simulink model "Astatic_StateSpace"  (R2021a)
settings: Solver=FixedStepAuto  StartTime=0.0  StopTime=STime  FixedStep=1e-3  RelTol=1e-3
undefined symbols (not defined in the file): C, J, Ka_, Kp, Mc, Ra, Ta, Tp, TPert
settings Model: Creator=akangmufti  LastModifiedBy=akangmufti

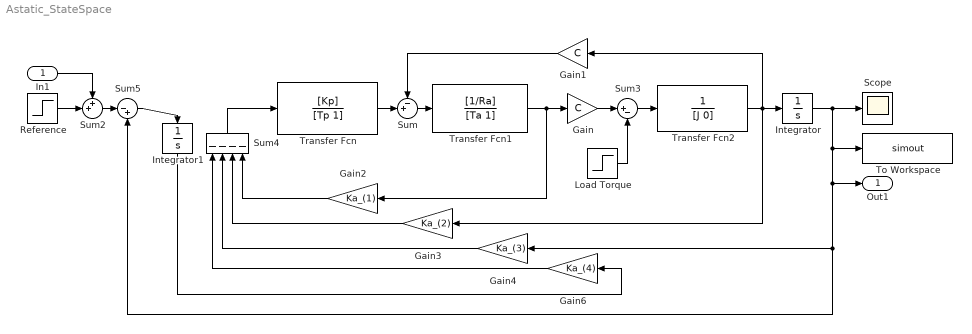
== system Astatic_StateSpace ==
  In1 : Inport
  Gain : Gain  Gain=C
  Gain1 : Gain  Gain=C
  Gain2 : Gain  Gain=Ka_(1)
  Gain3 : Gain  Gain=Ka_(2)
  Gain4 : Gain  Gain=Ka_(3)
  Gain6 : Gain  Gain=Ka_(4)
  Integrator : Integrator
  Integrator1 : Integrator
  Load Torque : Step  Time=TPert  After=Mc  SampleTime=0
  Reference : Step  Time=1e-3  SampleTime=0
  Scope : Scope
  Sum : Sum  Inputs=-+|
  Sum2 : Sum  Inputs=++|
  Sum3 : Sum  Inputs=|+-
  Sum4 : Sum  Inputs=----
  Sum5 : Sum  Inputs=|-+
  To Workspace : ToWorkspace  VariableName=simout  SampleTime=-1
  Transfer Fcn : TransferFcn  Numerator=[Kp]  Denominator=[Tp 1]
  Transfer Fcn1 : TransferFcn  Numerator=[1/Ra]  Denominator=[Ta 1]
  Transfer Fcn2 : TransferFcn  Denominator=[J 0]
  Out1 : Outport
  wires:
  Gain/1 -> Sum3/1
  Sum/1 -> Transfer Fcn1/1
  Transfer Fcn1/1 -> Gain2/1, Gain/1
  Transfer Fcn/1 -> Sum/2
  Gain1/1 -> Sum/1
  Sum3/1 -> Transfer Fcn2/1
  Transfer Fcn2/1 -> Gain3/1, Integrator/1, Gain1/1
  Load Torque/1 -> Sum3/2
  Gain3/1 -> Sum4/3
  Gain4/1 -> Sum4/2
  Gain2/1 -> Sum4/4
  Sum4/1 -> Transfer Fcn/1
  Integrator1/1 -> Gain6/1
  Sum5/1 -> Integrator1/1
  Gain6/1 -> Sum4/1
  In1/1 -> Sum2/1
  Integrator/1 -> Gain4/1, Sum5/2, Out1/1, To Workspace/1, Scope/1
  Sum2/1 -> Sum5/1
  Reference/1 -> Sum2/2
